simulink model "RBDEvaluation"  (R2021a)
settings: Solver=ode4  StartTime=0.0  StopTime=15  FixedStep=0.0015  RelTol=1e-3
undefined symbols (not defined in the file): F, L, m, X0
libraries: shared6dof x1
settings Model: Creator=User01  LastModifiedBy=User01

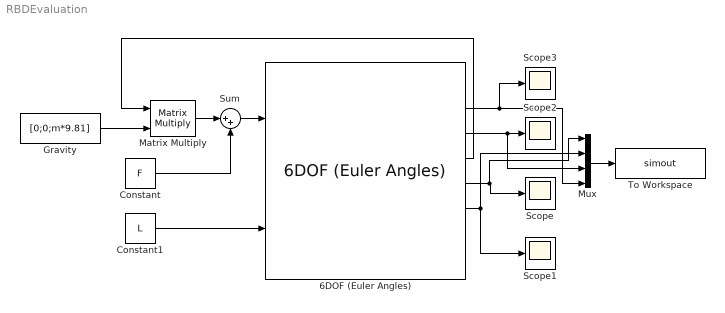
== system RBDEvaluation ==
  6DOF (Euler Angles) : shared6dof/6DOF (Euler Angles)  units=Metric (MKS)  mtype=Fixed  rep=Euler Angles  xme_0=X0(10:12)  Vm_0=X0(1:3)  eul_0=X0(7:9)  pm_0=X0(4:6)  mass_0=m  mass_e=0.5  mass_f=2.0  inertia=Inertia  inertia_e=eye(3)  inertia_f=2*eye(3)  k_quat=1.0  vre_flag=on  abi_flag=off  aMode=0  xme_statename=''  Vm_statename=''  eul_statename=''  quat_statename=''  pm_statename=''  mass_statename=''
      settings: SourceProductBaseCode=AE,PW,DR,MT,UV,VE
  Constant : Constant  Value=F
  Constant1 : Constant  Value=L
  Gravity : Constant  Value=[0;0;m*9.81]
  Matrix Multiply : Product  Multiplication=Matrix(*)
  Mux : Mux
  Scope{,1..3} (4 alike) : Scope
  Sum : Sum  Inputs=|++
  To Workspace : ToWorkspace  VariableName=simout  SaveFormat=Timeseries  SampleTime=-1
      settings: Save2DSignal=2-D array (concatenate along first dimension)
  wires:
  Constant/1 -> Sum/2
  6DOF (Euler Angles)/5 -> Mux/1, Scope/1
  6DOF (Euler Angles)/2 -> Mux/4, Scope3/1
  Gravity/1 -> Matrix Multiply/2
  Matrix Multiply/1 -> Sum/1
  6DOF (Euler Angles)/4 -> Matrix Multiply/1
  Sum/1 -> 6DOF (Euler Angles)/1
  6DOF (Euler Angles)/6 -> Scope1/1, Mux/2
  6DOF (Euler Angles)/3 -> Mux/3, Scope2/1
  Constant1/1 -> 6DOF (Euler Angles)/2
  Mux/1 -> To Workspace/1
